simulink model "fir_vergleich_1"  (Simulink 5.0)
settings: Solver=ode45  StartTime=0.0  StopTime=10.0  RelTol=1e-3
values from neighbouring files (symbols this model uses):
  frausch = 250    [analog_bp3.m]    (also in analog_tp2.m = 500)
  fs = 16000    [G722_1.m]    (also in TP_fdesign1.m = 0.215; adaptiv_2.m = 1000; adaptiv_3.m = 1000; adaptiv_4.m = 1000)
undefined symbols (not defined in the file or in its folder): bf, fpuls, fsin, ki
libraries: dsparch4 x1, dspsigops x1
settings Model: Creator=svenhoffmann  LastModifiedBy=svenhoffmann  ExtModeAutoUpdateStatusClock=off

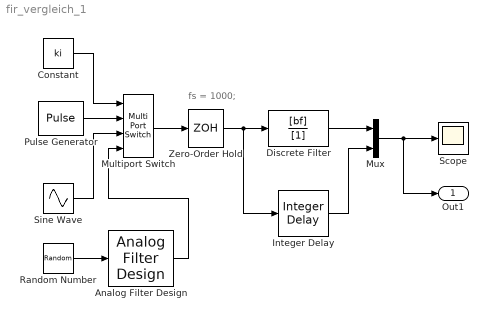
== system fir_vergleich_1 ==
  note: fs = 1000;
  Analog Filter Design : dsparch4/Analog Filter Design  method=Butterworth  filttype=Lowpass  N=8  Wlo=2*pi*frausch  Whi=80  Rp=2  Rs=40
  Constant : Constant  Value=ki
  Discrete Filter : DiscreteFilter  Numerator=[bf]  Denominator=[1]  SampleTime=1/fs
  Integer Delay : dspsigops/Integer Delay  delay=delay  ic=0  reset_popup=None
  Multiport Switch : MultiPortSwitch  Inputs=3  SaturateOnIntegerOverflow=on
  Mux : Mux  Inputs=2
  Pulse Generator : DiscretePulseGenerator  PulseType=Time based  Period=1/fpuls  PulseWidth=50
  Random Number : RandomNumber  SampleTime=0
  Scope : Scope
  Sine Wave : Sin  Frequency=2*pi*fsin  Samples=20  SampleTime=0
  Zero-Order Hold : ZeroOrderHold  SampleTime=1/fs
  Out1 : Outport
  wires:
  Discrete Filter/1 -> Mux/1
  Mux/1 -> Scope/1, Out1/1
  Integer Delay/1 -> Mux/2
  Multiport Switch/1 -> Zero-Order Hold/1
  Zero-Order Hold/1 -> Discrete Filter/1, Integer Delay/1
  Pulse Generator/1 -> Multiport Switch/2
  Sine Wave/1 -> Multiport Switch/3
  Random Number/1 -> Analog Filter Design/1
  Analog Filter Design/1 -> Multiport Switch/4
  Constant/1 -> Multiport Switch/1
